simulink model "e2b"  (R2021a)
settings: Solver=VariableStepAuto  StartTime=0.0  StopTime=10.0  RelTol=1e-3
undefined symbols (not defined in the file): Rec, SDTV
libraries: visionconversions x1, visionsources x1
settings Model: Creator=pranshu  LastModifiedBy=pranshu

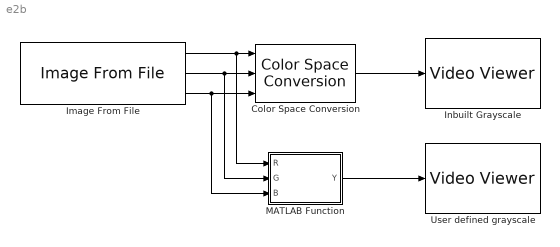
== system e2b ==
  Color Space Conversion : visionconversions/Color Space  Conversion  conversion=Obsolete  conversionActive=R'G'B' to intensity  wp_str=D65  rec=Rec. 601 (SDTV)  sys=1125/60/2:1  imagePorts=Separate color signals
  Image From File : visionsources/Image From File  Tag=vipblks_nd  FileName=peppers.png  Ts=inf  imagePorts=Separate color signals  OutPortLabels=R|G|B  ImageDataType=Inherit from input image  sdImageDataType=uint(8)  Signed=on  WordLength=16  FractionLengthMode=User-defined  FractionLength=15
  Inbuilt Grayscale : VideoViewer  FigPos=[1003.4 582.8 417.6 304]
  MATLAB Function : MATLAB Function  TreatAsAtomicUnit=on
  User defined grayscale : VideoViewer  FigPos=[477.8 583 417.6 304]
  wires:
  Color Space Conversion/1 -> Inbuilt Grayscale/1
  Image From File/1 -> MATLAB Function/1(R), Color Space Conversion/1
  Image From File/2 -> MATLAB Function/2(G), Color Space Conversion/2
  Image From File/3 -> MATLAB Function/3(B), Color Space Conversion/3
  MATLAB Function/1(Y) -> User defined grayscale/1

== matlab function e2b/MATLAB Function ==
  data: R input; Y output; G input; B input
function Y = fcn(R,G,B)
Y=0.2989*R+0.5870*G+0.1140*B;
